simulink model "stm32f0_mpl3115a2_demo"  (Simulink 7.3)
settings: Solver=ode3  SolverMode=SingleTasking  StartTime=0.0  StopTime=10.0  RelTol=1e-3
PreLoadFcn:
  | waijung.modelPreload; % Required for working with Waijung Blockset. Do not remove.
undefined symbols (not defined in the file): LQFP48, STM32F072CB
libraries: simulink x13, waijung_soft_i2c_lib x7, stm32f0_device_config_lib x1
CloseFcn:
  | waijung.modelClose; % Required for working with Waijung Blockset. Do not remove.
settings Model: Creator=Krisada  LastModifiedBy=Krisada
settings OptimizationCC: OptimizeModelRefInitCode=on  LifeSpan=1
settings HardwareCC: ProdEndianess=LittleEndian  ProdHWDeviceType=ARM Compatible->Cortex - M0  TargetEndianess=LittleEndian  TargetHWDeviceType=ARM Compatible->Cortex - M0
settings RTWCC: SystemTargetFile=stm32f0.tlc  GenerateMakefile=off  TemplateMakefile=ert_default_tmf  Description=STM32F0 Target  ProcessScript=stm32f0_make_rtw_hook
settings CodeAppCC: IgnoreCustomStorageClasses=off
settings STFCustomTargetCC: ModelReferenceCompliant=off  CombineOutputUpdateFcns=on  ERTCustomFileBanners=on  SupportContinuousTime=off  SupportNonInlinedSFcns=off  SystemTargetFile=stm32f0.tlc
settings ERTTargetCC: MultiwordLength=2048  ModelReferenceCompliant=off  ParMdlRefBuildCompliant=off  CompOptLevelCompliant=off  ERTFirstTimeCompliant=off  ModelStepFunctionPrototypeControlCompliant=off  CPPClassGenCompliant=off  InlinedParameterPlacement=NonHierarchical  ERTSrcFileBannerTemplate=stm32f0_code_template.cgt  ERTHdrFileBannerTemplate=stm32f0_code_template.cgt  ERTDataSrcFileTemplate=stm32f0_code_template.cgt  ERTDataHdrFileTemplate=stm32f0_code_template.cgt  ERTCustomFileTemplate=stm32f0_file_process.tlc

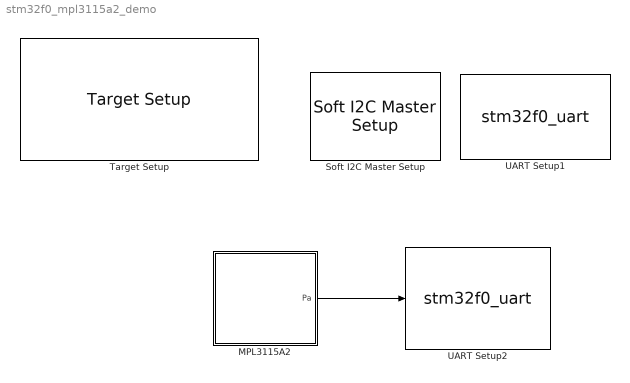
== system stm32f0_mpl3115a2_demo ==
  MPL3115A2 : Subsystem
  Soft I2C Master Setup : waijung_soft_i2c_lib/Soft I2C Master Setup  conf=Setup  targetname=stm32f0  module=1  transfer=Blocking  clk=250  timeout=25  sdapins='B7'  sclpins='B6'  writecount=1  readcount=1  waittime=0  forcestop=off  portpinstr=0  sampletime=-1  blockid=SoftI2CMasterSetup  inputporttype=[]  inputportwidth=[]  inputportlabel={}  outputporttype=[]  outputportwidth=[]  outputportlabel={}  compat=0  optionstring="[\"1\",\"250000\",\"3\",\"2\",\"1\",\"1\",\"25\",\"\",\"\",\"\",\"0\",\"1\",\"0\",\"0\",\"0\",\"0\",\"0\",\"0\",\"0\",\"\",\"1\",\"B\",\"7\",\"B\",\"6\"]"
  Target Setup : stm32f0_device_config_lib/Target Setup  Priority=100  compiler=GNU ARM  previous_compiler=GNU ARM  mcu=STM32F072CB (LQFP48)  mcustr=STM32F072CB  stdlib=STM32F072  clockconfig=FiO MOTE-ST Default (HSEOSC-8MHz/HCLK-48MHz)  system_stm32f0xx_c_path=F:\trunk\targets\stm32f0_target\stm32f0\utils\STM32F0xx_AN4055\stm32f0_default\hse8mhz_pll_hclk48mhz  showmemoryconfiguration=on  stacksize=0x400  heapsize=0x200  enableautocompiledownload=on  fullchiperase=off  programmerinterface=aMG USB Connect  editctrlstr=on  compilercontrolstr=$(patsubst %, -I%, .) -mcpu=cortex-m0 -mthumb -mabi=aapcs -Wall -O3 -mfloat-abi=soft -ffunction-sections -fdata-sections -fno-strict-aliasing -fno-builtin --short-enums  assemblercontrolstr=$(patsubst %, -I%, .) -mcpu=cortex-m0 -mtune=cortex-m0 -mthumb -Wall -O3 -Wa,-amhls=$(<:.s=.lst) -D__STACK_SIZE=$(STACK_SIZE) -D__HEAP_SIZE=$(HEAP_SIZE)  linkercontrolstr="-T$(LD_SCRIPT) -Wl,-Map=$(MAP),--cref,--no-warn-mismatch -mcpu=cortex-m0 -mthumb  -Wall -O3 -mabi=aapcs -lc -specs=nosys.specs"  runafterdownload=on  execprofile=None  profileruart=3  profilerbaud=500000  profilertxpin=Not used  profilerinitstr=0.1,48000000,4800000,500000,0  manualsetsampletime=off  sampletime=0.1  blockid=TargetSetup  systickreloadvalue=4800000  hseval=8000000  lastprofileruart=3  hclk=48000000  flashorigin=0x8000000  flashlength=128k  ramorigin=0x20000000  ramlength=16k  useextram=off
  UART Setup1 : S-Function  FunctionName=stm32f0_uart  Parameters=conf,inputporttype,inputportwidth,outputporttype,outputportwidth,asciiheader,optionstring,headerstring,terminatorstring,asciidatatypestring,sampletime,blockid  EnableBusSupport=off  mask(stm32f0_uart){conf=Setup, uartmodule=1, baudrate=115200, databits=8, parity=No, stopbit=1, remaptxpin=A9, remaprxpin=A10, flowcontrol=None, remapctspin=Not used, remaprtspin=Not used, advanceoptions=off, rxbuffersize=64, txbuffersize=64, transfer=Non-Blocking, packetmode=Binary, binheader='7E 7E', binterminator='03 03', porttype_double=1, porttype_single=1, porttype_int8=0, porttype_uint8=0, porttype_int16=0, porttype_uint16=1, porttype_int32=0, porttype_uint32=0, asciiformat='%1.2f', rx_asciiterminator=CR (0x0D - "\r"), tx_asciiterminator=CR (0x0D - "\r"), storagename=<empty>, varname=, asciiheader=, sampletime=-1, enablecustomportlabel=off, cinputportlabel=de, coutputportlabel=fff,ff,sdfsd, portpinstr=0, blockid=UARTSetup1, inputporttype=[], inputportwidth=[], inputportlabel={}, outputporttype=[], outputportwidth=[], outputportlabel={}, compat=0, optionstring=["1", "1", "A", "9", "1", "A", "10", "0", "*", "*", "0", "*", "*", "1", "1", "", "", "115200", "8", "No", "1", "None", "3", "2", "64", "64", "Binary", "Non-Blocking", ""], headerstring=[], terminatorstring=[], asciidatatypestring=[], lastmodule=1}
      mask prompts: conf "Configuration"; uartmodule "UART Module"; baudrate "Baud rate (bps)"; databits "Data bits"; stopbit "Stop bit"; remaptxpin "Tx pin"; remaprxpin "Rx pin"; flowcontrol "Hardware flow control"; remapctspin "HW Flow control, CTS Pin"; remaprtspin "HW Flow control, RTS Pin"; advanceoptions "Advance options"; rxbuffersize "Rx buffer size (bytes)"; txbuffersize "Tx buffer size (bytes)"; packetmode "Packet mode"; binheader "Binary header (example: '7E 7E')"; binterminator "Binary terminator (example: '03 03')"; porttype_double "Number of data port, type DOUBLE"; porttype_single "Number of data port, type SINGLE"; porttype_int8 "Number of data port, type INT8"; porttype_uint8 "Number of data port, type UINT8"; porttype_int16 "Number of data port, type INT16"; porttype_uint16 "Number of data port, type UINT16"; porttype_int32 "Number of data port, type INT32"; porttype_uint32 "Number of data port, type UINT32"; asciiformat "Ascii format"; rx_asciiterminator "End of packet"; tx_asciiterminator "End of packet"; storagename "Buffer"; varname "Var name"; asciiheader "Ascii header (printf format)"; sampletime "Sample time (sec)"; enablecustomportlabel "Enable custom port labels (Ex. In1, In2, In3)"; cinputportlabel "Custom input port labels (Ex. In1, In2, In3)"; coutputportlabel "Custom output port labels (Ex. Out1, Out2, Out3)"; portpinstr "Port Pin String"; blockid "Block ID"; inputporttype "Input Port Type"; inputportwidth "Input Port Width"; inputportlabel "Input Port Label"; outputporttype "Output Port Type"; outputportwidth "Output Port Width"; outputportlabel "Output port label"; compat "Compatibility (Reserved for future use)"; optionstring "String(s) to be passed to TLC"; lastmodule "Last module selected"
      mask init:
      | stm32f0_uart_callback('init');
      mask Help: web(fullfile(waijungdocroot,'stm32f0_uart.htm'), '-browser')
      mask StyleString: popup(Setup|Tx|Rx),popup(1|2|3|4),edit,popup(8),popup(No|Odd|Even),popup(0.5|1|1.5|2),popup(Not used|A9|B6),popup(Not used|A10|B7),popup(None|RTS|CTS|RTS/CTS),popup(Not used|A11),popup(Not used|A12),checkbox,popup(16|32|64|128|256|512),popup(16|32|64|128|256|512),popup(Blocking|Non-Blocking),popup(Ascii|Binary|String Buffer),edit,edit,edit,edit,edit,edit,edit,edit,edit,edit,edit,popup(CR (0x0D - "\r")|LF (0x0A - "\n")|CRLF (0x0D 0x0A - "\r\n")),popup(CR (0x0D - "\r")|LF (0x0A - "\n")|CRLF (0x0D 0x0A - "\r\n")|None),popup(<empty>),edit,edit,edit,checkbox,edit,edit,edit,edit,edit,edit,edit,edit,edit,edit,edit,edit,edit,edit,edit,edit
      mask CallbackString: stm32f0_uart_callback('conf');|stm32f0_uart_callback('uartmodule');|||||||stm32f0_uart_callback('flowcontrol');|||stm32f0_uart_callback('advanceoptions');|||stm32f0_uart_callback('conf');|stm32f0_uart_callback('conf');|stm32f0_uart_callback('binheader');|stm32f0_uart_callback('binterminator');|||||||||stm32f0_uart_callback('asciiformat');|||stm32f0_uart_callback('storagename');|||stm32f0_uart_callback('sampletime');|stm32f0_uart_callback('enablecustomportlabel');|stm32f0_uart_callback('conf');|stm32f0_uart_callback('conf');||stm32f0_uart_callback('blockid');||||||||||||
      mask Display: text(0.5, 0.5, 'Module: USART1_Setup\nBaud (Bps): 115200\nDMA Buffer: 64/64\nTx/Rx Pin: A9/A10','ver','middle','hor','center');
  UART Setup2 : S-Function  FunctionName=stm32f0_uart  Parameters=conf,inputporttype,inputportwidth,outputporttype,outputportwidth,asciiheader,optionstring,headerstring,terminatorstring,asciidatatypestring,sampletime,blockid  EnableBusSupport=off  mask(stm32f0_uart){conf=Tx, uartmodule=1, baudrate=115200, databits=8, parity=No, stopbit=1, remaptxpin=A9, remaprxpin=A10, flowcontrol=None, remapctspin=Not used, remaprtspin=Not used, advanceoptions=off, rxbuffersize=64, txbuffersize=64, transfer=Blocking, packetmode=Ascii, binheader='7E 7E', binterminator='03 03', porttype_double=1, porttype_single=1, porttype_int8=0, porttype_uint8=0, porttype_int16=0, porttype_uint16=1, porttype_int32=0, porttype_uint32=0, asciiformat='Pa=%1.2f', rx_asciiterminator=CR (0x0D - "\r"), tx_asciiterminator=CR (0x0D - "\r"), storagename=<empty>, varname=, asciiheader=Pa=%1.2f\r, sampletime=inf, enablecustomportlabel=off, cinputportlabel=de, coutputportlabel=fff,ff,sdfsd, portpinstr=0, blockid=UARTSetup2, inputporttype=[ -1], inputportwidth=[], inputportlabel={ '%f'}, outputporttype=[], outputportwidth=[], outputportlabel={}, compat=0, optionstring=["1", "1", "A", "9", "1", "A", "10", "0", "*", "*", "0", "*", "*", "1", "1", "", "", "115200", "8", "No", "1", "None", "3", "2", "64", "64", "Ascii", "Blocking", ""], headerstring=[], terminatorstring=["13"], asciidatatypestring=["float"], lastmodule=1}
      mask prompts: conf "Configuration"; uartmodule "UART Module"; baudrate "Baud rate (bps)"; databits "Data bits"; stopbit "Stop bit"; remaptxpin "Tx pin"; remaprxpin "Rx pin"; flowcontrol "Hardware flow control"; remapctspin "HW Flow control, CTS Pin"; remaprtspin "HW Flow control, RTS Pin"; advanceoptions "Advance options"; rxbuffersize "Rx buffer size (bytes)"; txbuffersize "Tx buffer size (bytes)"; packetmode "Packet mode"; binheader "Binary header (example: '7E 7E')"; binterminator "Binary terminator (example: '03 03')"; porttype_double "Number of data port, type DOUBLE"; porttype_single "Number of data port, type SINGLE"; porttype_int8 "Number of data port, type INT8"; porttype_uint8 "Number of data port, type UINT8"; porttype_int16 "Number of data port, type INT16"; porttype_uint16 "Number of data port, type UINT16"; porttype_int32 "Number of data port, type INT32"; porttype_uint32 "Number of data port, type UINT32"; asciiformat "Ascii format"; rx_asciiterminator "End of packet"; tx_asciiterminator "End of packet"; storagename "Buffer"; varname "Var name"; asciiheader "Ascii header (printf format)"; sampletime "Sample time (sec)"; enablecustomportlabel "Enable custom port labels (Ex. In1, In2, In3)"; cinputportlabel "Custom input port labels (Ex. In1, In2, In3)"; coutputportlabel "Custom output port labels (Ex. Out1, Out2, Out3)"; portpinstr "Port Pin String"; blockid "Block ID"; inputporttype "Input Port Type"; inputportwidth "Input Port Width"; inputportlabel "Input Port Label"; outputporttype "Output Port Type"; outputportwidth "Output Port Width"; outputportlabel "Output port label"; compat "Compatibility (Reserved for future use)"; optionstring "String(s) to be passed to TLC"; lastmodule "Last module selected"
      mask init:
      | stm32f0_uart_callback('init');
      mask Help: web(fullfile(waijungdocroot,'stm32f0_uart.htm'), '-browser')
      mask StyleString: popup(Setup|Tx|Rx),popup(1|2|3|4),edit,popup(8),popup(No|Odd|Even),popup(0.5|1|1.5|2),popup(Not used|A9|B6),popup(Not used|A10|B7),popup(None|RTS|CTS|RTS/CTS),popup(Not used|A11),popup(Not used|A12),checkbox,popup(16|32|64|128|256|512),popup(16|32|64|128|256|512),popup(Blocking|Non-Blocking),popup(Ascii|Binary|String Buffer),edit,edit,edit,edit,edit,edit,edit,edit,edit,edit,edit,popup(CR (0x0D - "\r")|LF (0x0A - "\n")|CRLF (0x0D 0x0A - "\r\n")),popup(CR (0x0D - "\r")|LF (0x0A - "\n")|CRLF (0x0D 0x0A - "\r\n")|None),popup(<empty>),edit,edit,edit,checkbox,edit,edit,edit,edit,edit,edit,edit,edit,edit,edit,edit,edit,edit,edit,edit,edit
      mask CallbackString: stm32f0_uart_callback('conf');|stm32f0_uart_callback('uartmodule');|||||||stm32f0_uart_callback('flowcontrol');|||stm32f0_uart_callback('advanceoptions');|||stm32f0_uart_callback('conf');|stm32f0_uart_callback('conf');|stm32f0_uart_callback('binheader');|stm32f0_uart_callback('binterminator');|||||||||stm32f0_uart_callback('asciiformat');|||stm32f0_uart_callback('storagename');|||stm32f0_uart_callback('sampletime');|stm32f0_uart_callback('enablecustomportlabel');|stm32f0_uart_callback('conf');|stm32f0_uart_callback('conf');||stm32f0_uart_callback('blockid');||||||||||||
      mask Display: text(0.95, 0.5, 'Module: USART1_Tx\nPacket: Ascii\nTransfer: Blocking\nTs (sec): 0.5','ver','middle','hor','right'); port_label('input', 1,'%f');
  wires:
  MPL3115A2/1(Pa) -> UART Setup2/1

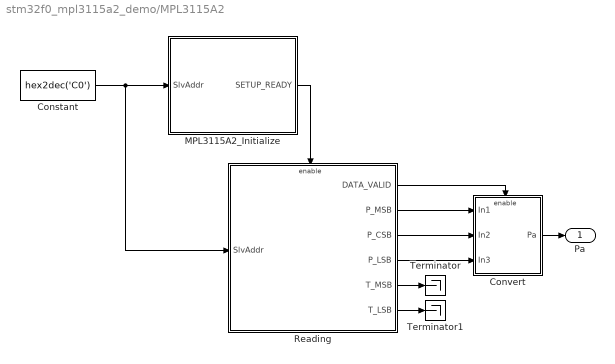
== system stm32f0_mpl3115a2_demo/MPL3115A2 ==
  Constant : Constant  Value=hex2dec('C0')  OutDataTypeMode=uint8  OutDataType=fixdt(1, 16)  OutScaling=2^0  OutDataTypeStr=uint8  SampleTime=0.5
  Convert : Subsystem
  MPL3115A2_Initialize : Subsystem
  Reading : Subsystem  TreatAsAtomicUnit=on
  Terminator : Terminator
  Terminator1 : Terminator
  Pa : Outport
  wires:
  Constant/1 -> MPL3115A2_Initialize/1(SlvAddr), Reading/1(SlvAddr)
  Reading/1(DATA_VALID) -> Convert/Enable
  Reading/6(T_LSB) -> Terminator1/1
  Reading/5(T_MSB) -> Terminator/1
  Reading/4(P_LSB) -> Convert/3(In3)
  Reading/3(P_CSB) -> Convert/2(In2)
  Reading/2(P_MSB) -> Convert/1(In1)
  MPL3115A2_Initialize/1(SETUP_READY) -> Reading/Enable
  Convert/1(Pa) -> Pa/1

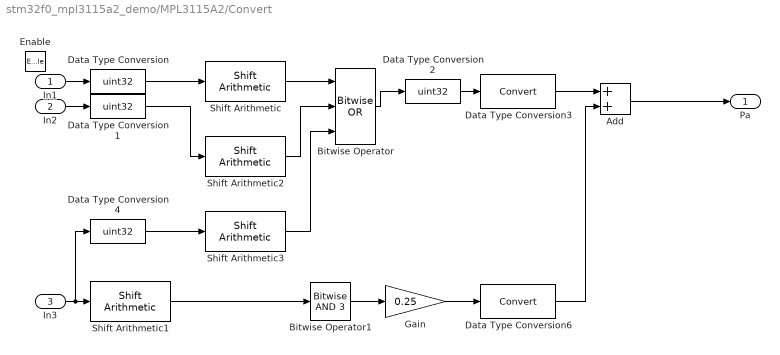
== system stm32f0_mpl3115a2_demo/MPL3115A2/Convert ==
  In1 : Inport
  In2 : Inport  Port=2
  In3 : Inport  Port=3
  Enable : EnablePort
  Add : Sum  OutDataType=fixdt(1, 16)  OutScaling=2^-10
  Bitwise Operator : simulink/Logic and Bit Operations/Bitwise Operator  logicop=OR  UseBitMask=off  NumInputPorts=3  BitMask=bin2dec('11011001')  BitMaskRealWorld=Stored Integer
  Bitwise Operator1 : simulink/Logic and Bit Operations/Bitwise Operator  logicop=AND  UseBitMask=on  BitMask=3  BitMaskRealWorld=Stored Integer
  Data Type Conversion{,1..2,4} (4 alike) : DataTypeConversion  OutDataTypeMode=uint32  OutDataType=fixdt(1, 16)  OutScaling=2^0  OutDataTypeStr=uint32
  Data Type Conversion3 : DataTypeConversion  OutDataType=fixdt(1, 16)  OutScaling=2^0
  Data Type Conversion6 : DataTypeConversion  OutDataType=fixdt(1, 16)  OutScaling=2^0
  Gain : Gain  Gain=0.25  ParameterDataType=fixdt(1, 16)  ParameterScaling=2^0  OutDataType=fixdt(1, 16)  OutScaling=2^0
  Shift Arithmetic : simulink/Logic and Bit Operations/Shift Arithmetic  SystemSampleTime=-1  nBitShiftRight=-10  nBinPtShiftRight=0
  Shift Arithmetic1 : simulink/Logic and Bit Operations/Shift Arithmetic  SystemSampleTime=-1  nBitShiftRight=4  nBinPtShiftRight=0
  Shift Arithmetic2 : simulink/Logic and Bit Operations/Shift Arithmetic  SystemSampleTime=-1  nBitShiftRight=-2  nBinPtShiftRight=0
  Shift Arithmetic3 : simulink/Logic and Bit Operations/Shift Arithmetic  SystemSampleTime=-1  nBitShiftRight=6  nBinPtShiftRight=0
  Pa : Outport  OutDataType=fixdt(1, 16)  OutScaling=2^0
  wires:
  Shift Arithmetic3/1 -> Bitwise Operator/3
  Data Type Conversion4/1 -> Shift Arithmetic3/1
  Shift Arithmetic2/1 -> Bitwise Operator/2
  In3/1 -> Data Type Conversion4/1, Shift Arithmetic1/1
  In2/1 -> Data Type Conversion1/1
  Add/1 -> Pa/1
  In1/1 -> Data Type Conversion/1
  Data Type Conversion6/1 -> Add/2
  Gain/1 -> Data Type Conversion6/1
  Data Type Conversion3/1 -> Add/1
  Bitwise Operator1/1 -> Gain/1
  Shift Arithmetic1/1 -> Bitwise Operator1/1
  Data Type Conversion2/1 -> Data Type Conversion3/1
  Bitwise Operator/1 -> Data Type Conversion2/1
  Data Type Conversion1/1 -> Shift Arithmetic2/1
  Shift Arithmetic/1 -> Bitwise Operator/1
  Data Type Conversion/1 -> Shift Arithmetic/1

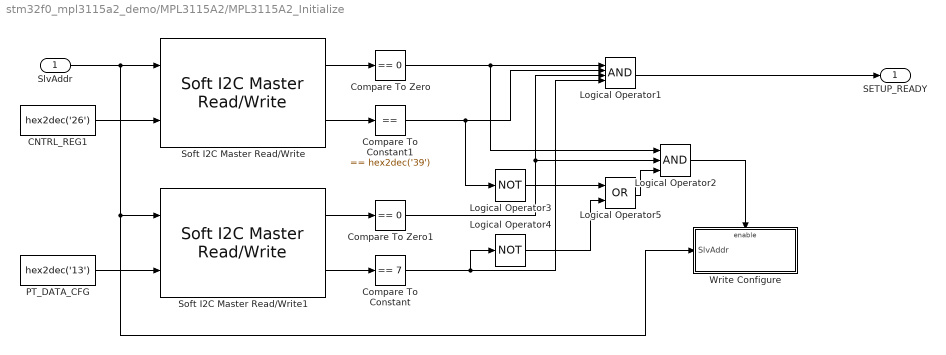
== system stm32f0_mpl3115a2_demo/MPL3115A2/MPL3115A2_Initialize ==
  SlvAddr : Inport  OutDataType=fixdt(1, 16)  OutScaling=2^0
  CNTRL_REG1 : Constant  Value=hex2dec('26')  OutDataTypeMode=uint8  OutDataType=fixdt(1, 16)  OutScaling=2^0  OutDataTypeStr=uint8
  Compare To Constant : simulink/Logic and Bit Operations/Compare To Constant  SystemSampleTime=-1  relop===  const=7  LogicOutDataTypeMode=boolean  ZeroCross=off
  Compare To Constant1 : simulink/Logic and Bit Operations/Compare To Constant  SystemSampleTime=-1  relop===  const=hex2dec('39')  LogicOutDataTypeMode=boolean  ZeroCross=off
  Compare To Zero : simulink/Logic and Bit Operations/Compare To Zero  SystemSampleTime=-1  relop===  LogicOutDataTypeMode=boolean  ZeroCross=off
  Compare To Zero1 : simulink/Logic and Bit Operations/Compare To Zero  SystemSampleTime=-1  relop===  LogicOutDataTypeMode=boolean  ZeroCross=off
  Logical Operator1 : Logic  Inputs=4  AllPortsSameDT=off  OutDataTypeMode=boolean  LogicDataType=fixdt(0, 8)  OutDataTypeStr=boolean
  Logical Operator2 : Logic  Inputs=3  AllPortsSameDT=off  OutDataTypeMode=boolean  LogicDataType=fixdt(0, 8)  OutDataTypeStr=boolean
  Logical Operator3 : Logic  Operator=NOT  Inputs=4  AllPortsSameDT=off  OutDataTypeMode=boolean  LogicDataType=fixdt(0, 8)  OutDataTypeStr=boolean
  Logical Operator4 : Logic  Operator=NOT  Inputs=4  AllPortsSameDT=off  OutDataTypeMode=boolean  LogicDataType=fixdt(0, 8)  OutDataTypeStr=boolean
  Logical Operator5 : Logic  Operator=OR  AllPortsSameDT=off  OutDataTypeMode=boolean  LogicDataType=fixdt(0, 8)  OutDataTypeStr=boolean
  PT_DATA_CFG : Constant  Value=hex2dec('13')  OutDataTypeMode=uint8  OutDataType=fixdt(1, 16)  OutScaling=2^0  OutDataTypeStr=uint8
  Soft I2C Master Read/Write : waijung_soft_i2c_lib/Soft I2C Master Read//Write  conf=ReadWrite  targetname=stm32f0  module=1  transfer=Blocking  clk=100  timeout=25  sdapins={'A4','A6'}  sclpins='A5'  writecount=1  readcount=1  waittime=0  forcestop=off  portpinstr=0  sampletime=inf  blockid=MPL3115A2MPL3115A2_InitializeSoftI2CMasterReadWrite  inputporttype=[3 3]  inputportwidth=[]  inputportlabel={'SlvAddr' 'Wr0 (uint8)'}  outputporttype=[3 3 ]  outputportwidth=[1 1]  outputportlabel={'Status' 'Rd0 (uint8)'}  compat=0  optionstring="[\"1\",\"1\",\"1\",\"0\",\"off\",\"1\"]"
  Soft I2C Master Read/Write1 : waijung_soft_i2c_lib/Soft I2C Master Read//Write  conf=ReadWrite  targetname=stm32f0  module=1  transfer=Blocking  clk=100  timeout=25  sdapins={'A4','A6'}  sclpins='A5'  writecount=1  readcount=1  waittime=0  forcestop=off  portpinstr=0  sampletime=inf  blockid=MPL3115A2MPL3115A2_InitializeSoftI2CMasterReadWrite1  inputporttype=[3 3]  inputportwidth=[]  inputportlabel={'SlvAddr' 'Wr0 (uint8)'}  outputporttype=[3 3 ]  outputportwidth=[1 1]  outputportlabel={'Status' 'Rd0 (uint8)'}  compat=0  optionstring="[\"1\",\"1\",\"1\",\"0\",\"off\",\"1\"]"
  Write Configure : Subsystem  TreatAsAtomicUnit=on
  SETUP_READY : Outport  OutDataType=fixdt(1, 16)  OutScaling=2^0
  wires:
  Logical Operator1/1 -> SETUP_READY/1
  Logical Operator5/1 -> Logical Operator2/3
  Logical Operator3/1 -> Logical Operator5/1
  Logical Operator4/1 -> Logical Operator5/2
  Logical Operator2/1 -> Write Configure/Enable
  Compare To Constant/1 -> Logical Operator4/1, Logical Operator1/4
  Compare To Zero1/1 -> Logical Operator2/2, Logical Operator1/3
  Compare To Constant1/1 -> Logical Operator3/1, Logical Operator1/2
  Soft I2C Master Read/Write/2 -> Compare To Constant1/1
  Soft I2C Master Read/Write1/2 -> Compare To Constant/1
  Compare To Zero/1 -> Logical Operator2/1, Logical Operator1/1
  Soft I2C Master Read/Write1/1 -> Compare To Zero1/1
  Soft I2C Master Read/Write/1 -> Compare To Zero/1
  PT_DATA_CFG/1 -> Soft I2C Master Read/Write1/2
  CNTRL_REG1/1 -> Soft I2C Master Read/Write/2
  SlvAddr/1 -> Write Configure/1(SlvAddr), Soft I2C Master Read/Write1/1, Soft I2C Master Read/Write/1

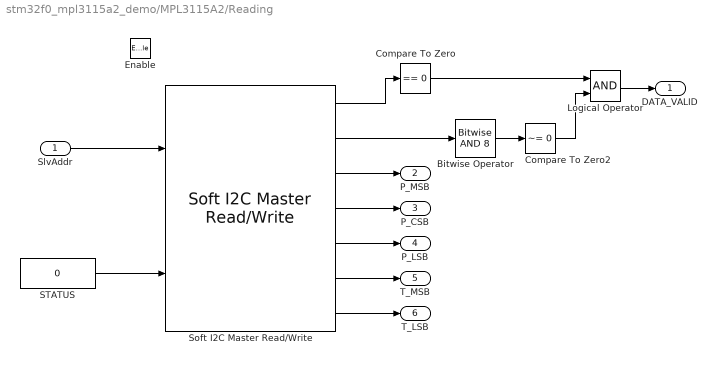
== system stm32f0_mpl3115a2_demo/MPL3115A2/Reading ==
  SlvAddr : Inport  OutDataType=fixdt(1, 16)  OutScaling=2^0
  Enable : EnablePort
  Bitwise Operator : simulink/Logic and Bit Operations/Bitwise Operator  logicop=AND  UseBitMask=on  BitMask=8  BitMaskRealWorld=Stored Integer
  Compare To Zero : simulink/Logic and Bit Operations/Compare To Zero  SystemSampleTime=-1  relop===  LogicOutDataTypeMode=boolean  ZeroCross=off
  Compare To Zero2 : simulink/Logic and Bit Operations/Compare To Zero  SystemSampleTime=-1  relop=~=  LogicOutDataTypeMode=boolean  ZeroCross=off
  Logical Operator : Logic  AllPortsSameDT=off  OutDataTypeMode=boolean  LogicDataType=fixdt(0, 8)  OutDataTypeStr=boolean
  STATUS : Constant  Value=0  OutDataTypeMode=uint8  OutDataType=fixdt(1, 16)  OutScaling=2^0  OutDataTypeStr=uint8
  Soft I2C Master Read/Write : waijung_soft_i2c_lib/Soft I2C Master Read//Write  conf=ReadWrite  targetname=stm32f0  module=1  transfer=Blocking  clk=100  timeout=25  sdapins={'A4','A6'}  sclpins='A5'  writecount=1  readcount=6  waittime=0  forcestop=off  portpinstr=0  sampletime=inf  blockid=MPL3115A2ReadingSoftI2CMasterReadWrite  inputporttype=[3 3]  inputportwidth=[]  inputportlabel={'SlvAddr' 'Wr0 (uint8)'}  outputporttype="[3 3 3 3 3 3 3      ]"  outputportwidth=[1 1 1 1 1 1 1]  outputportlabel={'Status' 'Rd0 (uint8)' 'Rd1 (uint8)' 'Rd2 (uint8)' 'Rd3 (uint8)' 'Rd4 (uint8)' 'Rd5 (uint8)'}  compat=0  optionstring="[\"1\",\"1\",\"6\",\"0\",\"off\",\"1\"]"
  DATA_VALID : Outport  OutDataType=fixdt(1, 16)  OutScaling=2^0
  P_MSB : Outport  Port=2  OutDataType=fixdt(1, 16)  OutScaling=2^0
  P_CSB : Outport  Port=3  OutDataType=fixdt(1, 16)  OutScaling=2^0
  P_LSB : Outport  Port=4  OutDataType=fixdt(1, 16)  OutScaling=2^0
  T_MSB : Outport  Port=5  OutDataType=fixdt(1, 16)  OutScaling=2^0
  T_LSB : Outport  Port=6  OutDataType=fixdt(1, 16)  OutScaling=2^0
  wires:
  Soft I2C Master Read/Write/7 -> T_LSB/1
  Soft I2C Master Read/Write/6 -> T_MSB/1
  Soft I2C Master Read/Write/5 -> P_LSB/1
  Soft I2C Master Read/Write/4 -> P_CSB/1
  Soft I2C Master Read/Write/3 -> P_MSB/1
  Compare To Zero/1 -> Logical Operator/1
  Soft I2C Master Read/Write/2 -> Bitwise Operator/1
  Soft I2C Master Read/Write/1 -> Compare To Zero/1
  Logical Operator/1 -> DATA_VALID/1
  Compare To Zero2/1 -> Logical Operator/2
  Bitwise Operator/1 -> Compare To Zero2/1
  STATUS/1 -> Soft I2C Master Read/Write/2
  SlvAddr/1 -> Soft I2C Master Read/Write/1

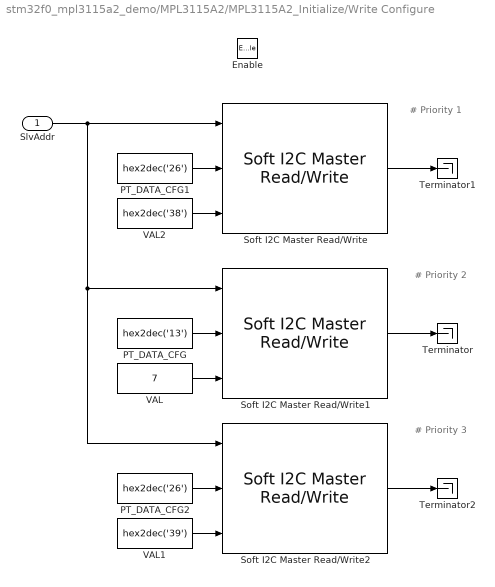
== system stm32f0_mpl3115a2_demo/MPL3115A2/MPL3115A2_Initialize/Write Configure ==
  note: # Priority 3
  note: # Priority 2
  note: # Priority 1
  SlvAddr : Inport  OutDataType=fixdt(1, 16)  OutScaling=2^0
  Enable : EnablePort
  PT_DATA_CFG : Constant  Value=hex2dec('13')  OutDataTypeMode=uint8  OutDataType=fixdt(1, 16)  OutScaling=2^0  OutDataTypeStr=uint8
  PT_DATA_CFG1 : Constant  Value=hex2dec('26')  OutDataTypeMode=uint8  OutDataType=fixdt(1, 16)  OutScaling=2^0  OutDataTypeStr=uint8
  PT_DATA_CFG2 : Constant  Value=hex2dec('26')  OutDataTypeMode=uint8  OutDataType=fixdt(1, 16)  OutScaling=2^0  OutDataTypeStr=uint8
  Soft I2C Master Read/Write : waijung_soft_i2c_lib/Soft I2C Master Read//Write  conf=ReadWrite  targetname=stm32f0  module=1  transfer=Blocking  clk=100  timeout=25  sdapins={'A4','A6'}  sclpins='A5'  writecount=2  readcount=0  waittime=0  forcestop=off  portpinstr=0  sampletime=inf  blockid=MPL3115A2MPL3115A2_InitializeWriteConfigureSoftI2CMasterReadWrite  inputporttype=[3 3 3]  inputportwidth=[]  inputportlabel={'SlvAddr' 'Wr0 (uint8)' 'Wr1 (uint8)'}  outputporttype=[3]  outputportwidth=[1]  outputportlabel={'Status'}  compat=0  optionstring="[\"1\",\"2\",\"0\",\"0\",\"off\",\"1\"]"
  Soft I2C Master Read/Write1 : waijung_soft_i2c_lib/Soft I2C Master Read//Write  conf=ReadWrite  targetname=stm32f0  module=1  transfer=Blocking  clk=100  timeout=25  sdapins={'A4','A6'}  sclpins='A5'  writecount=2  readcount=0  waittime=0  forcestop=off  portpinstr=0  sampletime=inf  blockid=MPL3115A2MPL3115A2_InitializeWriteConfigureSoftI2CMasterReadWrite1  inputporttype=[3 3 3]  inputportwidth=[]  inputportlabel={'SlvAddr' 'Wr0 (uint8)' 'Wr1 (uint8)'}  outputporttype=[3]  outputportwidth=[1]  outputportlabel={'Status'}  compat=0  optionstring="[\"1\",\"2\",\"0\",\"0\",\"off\",\"1\"]"
  Soft I2C Master Read/Write2 : waijung_soft_i2c_lib/Soft I2C Master Read//Write  conf=ReadWrite  targetname=stm32f0  module=1  transfer=Blocking  clk=100  timeout=25  sdapins={'A4','A6'}  sclpins='A5'  writecount=2  readcount=0  waittime=0  forcestop=off  portpinstr=0  sampletime=inf  blockid=MPL3115A2MPL3115A2_InitializeWriteConfigureSoftI2CMasterReadWrite2  inputporttype=[3 3 3]  inputportwidth=[]  inputportlabel={'SlvAddr' 'Wr0 (uint8)' 'Wr1 (uint8)'}  outputporttype=[3]  outputportwidth=[1]  outputportlabel={'Status'}  compat=0  optionstring="[\"1\",\"2\",\"0\",\"0\",\"off\",\"1\"]"
  Terminator : Terminator
  Terminator1 : Terminator
  Terminator2 : Terminator
  VAL : Constant  Value=7  OutDataTypeMode=uint8  OutDataType=fixdt(1, 16)  OutScaling=2^0  OutDataTypeStr=uint8
  VAL1 : Constant  Value=hex2dec('39')  OutDataTypeMode=uint8  OutDataType=fixdt(1, 16)  OutScaling=2^0  OutDataTypeStr=uint8
  VAL2 : Constant  Value=hex2dec('38')  OutDataTypeMode=uint8  OutDataType=fixdt(1, 16)  OutScaling=2^0  OutDataTypeStr=uint8
  wires:
  Soft I2C Master Read/Write2/1 -> Terminator2/1
  VAL1/1 -> Soft I2C Master Read/Write2/3
  PT_DATA_CFG2/1 -> Soft I2C Master Read/Write2/2
  Soft I2C Master Read/Write/1 -> Terminator1/1
  VAL2/1 -> Soft I2C Master Read/Write/3
  PT_DATA_CFG1/1 -> Soft I2C Master Read/Write/2
  Soft I2C Master Read/Write1/1 -> Terminator/1
  VAL/1 -> Soft I2C Master Read/Write1/3
  SlvAddr/1 -> Soft I2C Master Read/Write1/1, Soft I2C Master Read/Write2/1, Soft I2C Master Read/Write/1
  PT_DATA_CFG/1 -> Soft I2C Master Read/Write1/2
